simulink model "with_sssc"  (Simulink 7.3)
settings: Solver=FixedStepDiscrete  SolverMode=SingleTasking  StartTime=0.0  StopTime=0.8  FixedStep=Ts  RelTol=1e-3
PreLoadFcn:
  | Ts=1/512/60;
undefined symbols (not defined in the file): DiscIntNeverNeededParam
libraries: powerlib x54, powerlib_extras x38, simulink_extras x2, simulink x1
(part 1 of 7)
Description:
  | Copyright 2008-2009 The MathWorks(TM), Inc.
settings Model: Creator=Giroux/Sybille  LastModifiedBy=Bharath  ExtModeTrigMode=oneshot  ExtModeArmWhenConnect=off  ExtModeAutoUpdateStatusClock=off
settings DataIOCC: InitialState=xInitial_upfc  LimitDataPoints=off  SaveFinalState=on  SaveFormat=Structure  SaveOutput=off  SaveTime=off  SignalLoggingName=sigsOut
settings OptimizationCC: BlockReduction=off  BooleanDataType=off  InitFltsAndDblsToZero=on  EfficientMapNaN2IntZero=off
settings DebuggingCC: SignalResolutionControl=TryResolveAllWithWarning  SolverPrmCheckMsg=none  MultiTaskDSMMsg=warning  MultiTaskCondExecSysMsg=none  StrictBusMsg=None
settings HardwareCC: TargetEndianess=LittleEndian  TargetHWDeviceType=MATLAB Host  ProdEqTarget=off
settings RTWCC: SystemTargetFile=accel.tlc  TemplateMakefile=accel_default_tmf  ProcessScript=accel_make_rtw_hook  IncludeERTFirstTime=on
settings STFCustomTargetCC: SystemTargetFile=accel.tlc

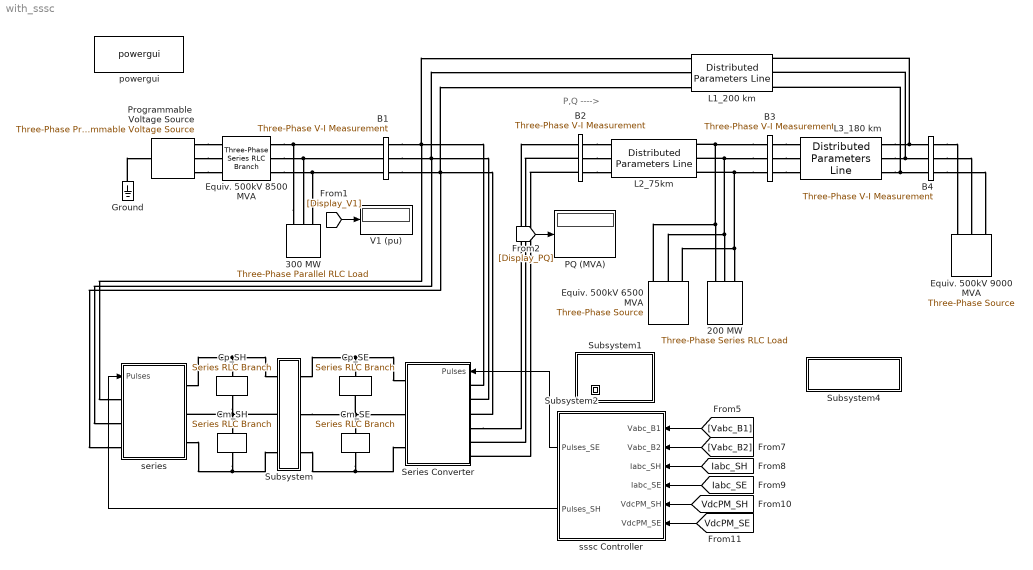
== system with_sssc ==
  note: P,Q
      | ---->
  200 MW : powerlib/Elements/Three-Phase Series RLC Load  DialogController=POWERSYS.PowerSysDialog  PhysicalDomain=powersysdomain  SubClassName=unknown  LeftPortType=p1  RightPortType=p1  LConnTagsString=A|B|C  Configuration=Y (grounded)  NominalVoltage=500e3  NominalFrequency=60  ActivePower=200e6  InductivePower=0  CapacitivePower=0  Measurements=None
  300 MW : powerlib/Elements/Three-Phase Parallel RLC Load  DialogController=POWERSYS.PowerSysDialog  PhysicalDomain=powersysdomain  SubClassName=unknown  LeftPortType=p1  RightPortType=p1  LConnTagsString=A|B|C  Configuration=Y (grounded)  NominalVoltage=500e3  NominalFrequency=60  ActivePower=300e6  InductivePower=0  CapacitivePower=0  Measurements=None
  B1 : powerlib/Measurements/Three-Phase V-I Measurement  DialogController=POWERSYS.PowerSysDialog  SystemSampleTime=-1  VoltageMeasurement=phase-to-ground  SetLabelV=on  LabelV=Vabc_B1  Vpu=on  CurrentMeasurement=yes  SetLabelI=on  LabelI=Iabc_B1  Ipu=on  Pbase=100e6  Vbase=500e3  OutputType=Magnitude  PhasorSimulation=off  PSBequivalent=0
  B2 : powerlib/Measurements/Three-Phase V-I Measurement  DialogController=POWERSYS.PowerSysDialog  SystemSampleTime=-1  VoltageMeasurement=phase-to-ground  SetLabelV=on  LabelV=Vabc_B2  Vpu=on  CurrentMeasurement=yes  SetLabelI=on  LabelI=Iabc_B2  Ipu=on  Pbase=100e6  Vbase=500e3  OutputType=Magnitude  PhasorSimulation=off  PSBequivalent=0
  B3 : powerlib/Measurements/Three-Phase V-I Measurement  DialogController=POWERSYS.PowerSysDialog  SystemSampleTime=-1  VoltageMeasurement=phase-to-ground  SetLabelV=on  LabelV=Vabc_B3  Vpu=on  CurrentMeasurement=yes  SetLabelI=on  LabelI=Iabc_B3  Ipu=on  Pbase=100e6  Vbase=500e3  OutputType=Magnitude  PhasorSimulation=off  PSBequivalent=0
  B4 : powerlib/Measurements/Three-Phase V-I Measurement  DialogController=POWERSYS.PowerSysDialog  SystemSampleTime=-1  VoltageMeasurement=phase-to-ground  SetLabelV=on  LabelV=Vabc_B4  Vpu=on  CurrentMeasurement=no  SetLabelI=on  LabelI=Iabc_B4  Ipu=on  Pbase=100e6  Vbase=500e3  OutputType=Magnitude  PhasorSimulation=off  PSBequivalent=0
  Cm_SE : powerlib/Elements/Series RLC Branch  DialogController=POWERSYS.PowerSysDialog  PhysicalDomain=powersysdomain  SubClassName=unknown  LeftPortType=p1  RightPortType=p1  LConnTagsString=__new0  RConnTagsString=__new0  BranchType=C  Resistance=1.0  Inductance=1.0  SetiL0=off  InitialCurrent=0  Capacitance=2500e-6  Setx0=off  InitialVoltage=0  Measurements=Branch voltage
  Cm_SH : powerlib/Elements/Series RLC Branch  DialogController=POWERSYS.PowerSysDialog  PhysicalDomain=powersysdomain  SubClassName=unknown  LeftPortType=p1  RightPortType=p1  LConnTagsString=__new0  RConnTagsString=__new0  BranchType=C  Resistance=1.0  Inductance=1.0  SetiL0=off  InitialCurrent=0  Capacitance=2500e-6  Setx0=off  InitialVoltage=0  Measurements=Branch voltage
  Cp_SE : powerlib/Elements/Series RLC Branch  DialogController=POWERSYS.PowerSysDialog  PhysicalDomain=powersysdomain  SubClassName=unknown  LeftPortType=p1  RightPortType=p1  LConnTagsString=__new0  RConnTagsString=__new0  BranchType=C  Resistance=1.0  Inductance=1.0  SetiL0=off  InitialCurrent=0  Capacitance=2500e-6  Setx0=off  InitialVoltage=0  Measurements=Branch voltage
  Cp_SH : powerlib/Elements/Series RLC Branch  DialogController=POWERSYS.PowerSysDialog  PhysicalDomain=powersysdomain  SubClassName=unknown  LeftPortType=p1  RightPortType=p1  LConnTagsString=__new0  RConnTagsString=__new0  BranchType=C  Resistance=1.0  Inductance=1.0  SetiL0=off  InitialCurrent=0  Capacitance=2500e-6  Setx0=off  InitialVoltage=0  Measurements=Branch voltage
  Equiv. 500kV 6500 MVA : powerlib/Electrical Sources/Three-Phase Source  DialogController=POWERSYS.PowerSysDialog  SystemSampleTime=-1  Voltage=500e3*1.00  PhaseAngle=9.2-20  Frequency=60  InternalConnection=Yg  SpecifyImpedance=on  Resistance=0.8929  Inductance=16.58e-3  ShortCircuitLevel=6500e6  BaseVoltage=500e3  XRratio=8
  "Equiv. 500kV 8500 MVA " : powerlib/Elements/Three-Phase Series RLC Branch  DialogController=POWERSYS.PowerSysDialog  PhysicalDomain=powersysdomain  SubClassName=unknown  LeftPortType=p1  RightPortType=p1  LConnTagsString=A|B|C  RConnTagsString=A|B|C  BranchType=RL  Resistance=500e3^2/8500e6/10  Inductance=500e3^2/8500e6/(2*pi*60)  Capacitance=1.0  Measurements=None
  Equiv. 500kV 9000 MVA : powerlib/Electrical Sources/Three-Phase Source  DialogController=POWERSYS.PowerSysDialog  SystemSampleTime=-1  Voltage=500e3*0.98  PhaseAngle=9.2-40  Frequency=60  InternalConnection=Yg  SpecifyImpedance=on  Resistance=0.8929  Inductance=16.58e-3  ShortCircuitLevel=9000e6  BaseVoltage=500e3  XRratio=10
  Ground : powerlib/Elements/Ground  DialogController=POWERSYS.PowerSysDialog  PhysicalDomain=powersysdomain  SubClassName=unknown  LeftPortType=p1  RightPortType=p1  LConnTagsString=a
  L1_200 km : powerlib/Elements/Distributed Parameters Line  DialogController=POWERSYS.PowerSysDialog  SystemSampleTime=-1  Phases=3  Frequency=60  Resistance=[0.01273*2 0.3864]  Inductance="[0.9337e-3  4.1264e-3]"  Capacitance=[12.74e-9 7.751e-9]  Length=200  x1=[0 -1.91503257172238e-010 88662.5919859554 -491984.755570925;0.000226216626798297 -1.96856066781718e-010 130246.803325563 -482644.615794399;0.000452433253596594 -2.0077801734948e-010 170884.308682266 -469796.347344288;0.000678649880394891 -2.03240601964242e-010 210279.732135357 -453533.338559508;0.000904866507193188 -2.04225921195624e-010 248146.725904086 -433973.798005056;0.00113108313399149 -2.03726813197136e-010 284210.051682097 -411259.895266619]  x2=[0 -4.21310497148667e-011 -44308.1155382362 -490501.124647627;0.000226216626798297 -3.40783030710814e-011 -2367.02497623426 -492492.598498595;0.000452433253596594 -2.57778564256003e-011 39591.27043571 -490904.363077395;0.000678649880394891 -1.72900420268886e-011 81261.7945424455 -485747.962559677;0.000904866507193188 -8.6765540161297e-012 122341.662870224 -477060.87652341;0.00113108313399149 0 162532.284158993 -464906.247526527]  x3=[0 -1.46364700661107e-012 -25.746556881283 50.0156886130386;0.000226216626798297 -1.43300403371694e-012 -29.9132391703324 47.6408692302741;0.000452433253596594 -1.39194519296574e-012 -33.8624954514681 44.9197695951003;0.000678649880394891 -1.34076892277742e-012 -37.5656203403433 41.8721681684003;0.000904866507193188 -1.27984720065879e-012 -40.9956974720401 38.5202166071091;0.00113108313399149 -1.20962283946473e-012 -44.1277951441326 34.8882787536893]  x4=[0 1.64774342243962e-013 -282.830205301423 -3649.3225183874;0.000226216626798297 4.44601431824641e-014 29.0408455107673 -3660.15087087025;0.000452433253596594 -7.61772168509498e-014 340.700811355867 -3644.37521742502;0.000678649880394891 -1.96260878635252e-013 649.884374799866 -3602.1102242479;0.000904866507193188 -3.1491800753529e-013 954.344218274468 -3533.66309674343;0.00113108313399149 -4.31286137747869e-013 1251.86735882721 -3439.53134658535]  x5=0.00113108313399149  Measurements=None
      settings: AttributesFormatString=\n
  L2_75km : powerlib/Elements/Distributed Parameters Line  DialogController=POWERSYS.PowerSysDialog  SystemSampleTime=-1  Phases=3  Frequency=60  Resistance=[0.01273*2 0.3864]  Inductance="[0.9337e-3  4.1264e-3]"  Capacitance=[12.74e-9 7.751e-9]  Length=75  x1=[0 -3.96693010864502e-010 167104.032532242 -471154.023466305;8.48312350493614e-005 -3.93822769631872e-010 182083.816625282 -465569.925188681;0.000169662470098723 -3.90549776474901e-010 196877.388510213 -459509.701105888;0.000254493705148084 -3.86877378595412e-010 211469.619200078 -452979.548845638;0.000339324940197445 -3.82809331655663e-010 225845.585614131 -445986.146618518;0.000424156175246807 -3.78349795937538e-010 239990.585839268 -438536.646388359]  x2=[0 -6.95097933782165e-012 120539.216595689 -484658.49781756;8.48312350493614e-005 -5.56933300650617e-012 135974.618856574 -480556.412163115;0.000169662470098723 -4.18199106854061e-012 151270.963542253 -475962.874427486;0.000254493705148084 -2.79037232110564e-012 166412.607493587 -470882.582297819;0.000339324940197445 -1.3958999351596e-012 181384.065759707 -465320.731251848;0.000424156175246807 0 196170.027434053 -459283.009244626]  x3=[0 4.40693316305242e-013 -104.937683284578 -46.5969347149227;8.48312350493614e-005 5.09069305089187e-013 -103.394079857967 -49.9285083723259;0.000169662470098723 5.769246824254e-013 -101.744738094624 -53.2090214908851;0.000254493705148084 6.44190054449671e-013 -99.991344731884 -56.4351191783158;0.000339324940197445 7.10796630680306e-013 -98.1356929178462 -59.603502191527;0.000424156175246807 7.76676294368304e-013 -96.1796803775706 -62.7109303106685]  x4=[0 -2.3638910297891e-012 990.165268579737 -3517.07349521636;8.48312350493614e-005 -2.47594506765685e-012 1102.11798749276 -3483.61438329502;0.000169662470098723 -2.58546702328494e-012 1212.94360006623 -3446.59267290369;0.000254493705148084 -2.69234489152335e-012 1322.52876793534 -3406.04622514705;0.000339324940197445 -2.79646937125895e-012 1430.76142130464 -3362.0165057836;0.000424156175246807 -2.89773397719475e-012 1537.53087355877 -3314.54854281976]  x5=0.000424156175246807  Measurements=None
      settings: AttributesFormatString=\n
  L3_180 km : powerlib/Elements/Distributed Parameters Line  DialogController=POWERSYS.PowerSysDialog  SystemSampleTime=-1  Phases=3  Frequency=60  Resistance=[0.01273*2 0.3864]  Inductance="[0.9337e-3  4.1264e-3]"  Capacitance=[12.74e-9 7.751e-9]  Length=180  x1=[0 -1.63454333087056e-011 53455.4761104332 -496554.200785859;0.000203594964118467 -1.31933594894557e-011 91372.9576361359 -490993.426490723;0.000407189928236935 -9.96360043581722e-012 128752.41625445 -482541.581164688;0.000610784892355402 -6.6751736383164e-012 165373.753967862 -471248.431024288;0.000814379856473869 -3.34744203531157e-012 201021.336751836 -457180.472477534;0.00101797482059234 0 235485.264252623 -440420.540579284]  x2=[0 -3.81393443869797e-011 -31539.306669084 -491487.369642364;0.000203594964118467 -3.07845054753967e-011 6239.89303884498 -492458.75575321;0.000407189928236935 -2.32484010169069e-011 43982.3509636315 -490530.442670838;0.000610784892355402 -1.55754051560716e-011 81465.8316926323 -485713.78470223;0.000814379856473869 -7.81069808239367e-012 118469.624724594 -478037.143327535;0.00101797482059234 0 154775.844058816 -467545.720201797]  x3=[0 -5.49396821505064e-013 -34.7229837874336 -492.811835812092;0.000203594964118467 -5.26694805439027e-013 3.16714661805268 -494.023441044943;0.000407189928236935 -5.0089150122538e-013 41.038628208007 -492.326133893369;0.000610784892355402 -4.72138844065877e-013 78.6684658517113 -487.729908453567;0.000814379856473869 -4.40606135563534e-013 115.835087268073 -480.261828253281;0.00101797482059234 -4.06479046839711e-013 152.319647689125 -469.965866896147]  x4=[0 9.1315487305108e-014 -310.779746226165 -3120.093262722;0.000203594964118467 7.3706094431248e-014 -70.6217835689112 -3134.73740246822;0.000407189928236935 5.56627048011912e-014 169.952014783101 -3130.92355885908;0.000610784892355402 3.72915616317389e-014 409.52510045736 -3108.674188596;0.000814379856473869 1.87008380204443e-014 646.686817484955 -3068.12030058126;0.00101797482059234 1.26217744835362e-029 880.040708535207 -3009.50068451039]  x5=0.00101797482059234  Measurements=None
      settings: AttributesFormatString=\n
  PQ (MVA) : Display
      settings: Format=bank  SampleTime=Ts*100
  Programmable  Voltage Source : powerlib/Electrical Sources/Three-Phase Programmable Voltage Source  DialogController=POWERSYS.PowerSysDialog  SystemSampleTime=-1  PositiveSequence="[500e3*1.0491 9.2  60]"  VariationEntity=None  VariationType=Modulation  VariationStep=-0.3  VariationRate=0.5  VariationMagnitude=0.4  VariationFrequency=2  VariationTiming=[0.1 1.2]  VariationPhaseA=off  Amplitudes="[1  0.8  1.2  1.0 ]"  TimeValues=[0 0.1 0.25 0.4]  HarmonicGeneration=off  HarmonicA=[3 0.2 -25 0]  HarmonicB="[2 0.15  35 2]"  Timing="[0.1  0.6]"
  Series Converter : Subsystem
  Subsystem : Subsystem
      mask Display: disp('Sw')
  Subsystem1 : Subsystem  mask(UPFC GUI){OpMode=SSSC (Voltage Injection), Par_VarControl=[0.3  0.5  +0.8  -0.8 ], Par_Vref=[ 1  1.005  0.3 *100], Par_SSSC=[ 0.0  0.08  0.3  ], Par_UPFC_Pref=[  +8.7  +10   0.25  ], Par_UPFC_Qref=[  -0.6  +0.7  0.5  ]}
      mask prompts: OpMode "Operation Mode:"; Par_VarControl "STATCOM (Qref): [T1 T2 Q1 Q2]"; Par_Vref "STATCOM Vref (pu): [ Initial   Final  StepTime ]"; Par_SSSC "SSSC Votage Injection (pu): [ Initial  Final  StepTime ]"; Par_UPFC_Pref "UPFC Pref (pu): [ Initial  Final  StepTime ]"; Par_UPFC_Qref "UPFC Qref (pu): [ Initial  Final  StepTime ]"
      mask StyleString: popup(STATCOM (Var Control)|STATCOM (Voltage Control)|SSSC (Voltage Injection)|STATCOM  (Voltage Control) + SSSC (Voltage Injection)|UPFC  (Power Flow Control)),edit,edit,edit,edit,edit
      mask Display: disp('SSSC\nGUI')
  Subsystem2 : Subsystem  mask(UPFC GUI){OpMode=SSSC (Voltage Injection), Par_VarControl=[0.05 0.15 -0.5 0.5]*100, Par_Vref=[ 1  1.005  0.1*100 ], Par_SSSC=[ 0.0  0.08 0.1*100 ], Par_UPFC_Pref=[  8.7  10  0.1*100 ], Par_UPFC_Qref=[  -0.6  +0.5  0.1*100 ]}
      mask prompts: OpMode "Operation Mode:"; Par_VarControl "STATCOM (Qref): [T1 T2 Q1 Q2]"; Par_Vref "STATCOM Vref (pu): [ Initial   Final  StepTime ]"; Par_SSSC "SSSC Votage Injection (pu): [ Initial  Final  StepTime ]"; Par_UPFC_Pref "UPFC Pref (pu): [ Initial  Final  StepTime ]"; Par_UPFC_Qref "UPFC Qref (pu): [ Initial  Final  StepTime ]"
      settings: OpenFcn=openfig('power_upfc_gto48p_PQregion.fig');
      mask StyleString: popup(STATCOM (Var Control)|STATCOM (Voltage Control)|SSSC (Voltage Injection)|STATCOM  (Voltage Control) + SSSC (Voltage Injection)|UPFC  (Power Flow Control)),edit,edit,edit,edit,edit
      mask Display: disp('Show UPFC\nControllable Region')
  Subsystem4 : Subsystem
      mask Display: disp('Show Scopes')
  V1 (pu) : Display
      settings: Format=bank  SampleTime=Ts*100
  powergui : powerlib/powergui  Priority=2  SystemSampleTime=-1  SimulationMode=Discrete  SampleTime=Ts  frequency=60  SPID=off  DisableSnubberDevices=off  DisableRonSwitches=off  DisableVfSwitches=off  SwTol=0  Interpol=off  frequencyindice=60  echomessages=off  HookPort=off  DisplayEquations=off  FunctionMessages=off  EnableUseOfTLC=off  x0status=blocks  RestoreLinks=yes  Frange=[0:2:500]  Ylog=off  Xlog=on  ShowGrid=off  save=off  variable=ZData  ZoomFFT=on  StartTime=0.0  cycles=1  DisplayStyle=1  fundamental=60  FreqAxis=off  MaxFrequency=1000  frequencyindicesteady=1  RmsSteady=1  display=off  Ts=0  methode=off
  series : Subsystem
  sssc Controller : Subsystem
  wires:
  [Vabc_B1] -> sssc Controller/1(Vabc_B1)
  [Vabc_B2] -> sssc Controller/2(Vabc_B2)
  [Iabc_SH] -> sssc Controller/3("Iabc_SH ")
  [Iabc_SE] -> sssc Controller/4(Iabc_SE)
  [VdcPM_SH] -> sssc Controller/5("VdcPM_SH ")
  [VdcPM_SE] -> sssc Controller/6(VdcPM_SE)
  sssc Controller/2(Pulses_SH) -> series/1(Pulses)
  sssc Controller/1(Pulses_SE) -> Series Converter/1(Pulses)
  [Display_V1] -> V1 (pu)/1
  [Display_PQ] -> PQ (MVA)/1
  connections:
  Ground/LConn1 -- Programmable  Voltage Source/LConn1
  Programmable  Voltage Source/RConn1 -- "Equiv. 500kV 8500 MVA "/LConn1
  Programmable  Voltage Source/RConn2 -- "Equiv. 500kV 8500 MVA "/LConn2
  Programmable  Voltage Source/RConn3 -- "Equiv. 500kV 8500 MVA "/LConn3
  Subsystem/LConn2 -- series/RConn2 -- Cp_SH/RConn1 -- Cm_SH/LConn1
  Subsystem/RConn3 -- Series Converter/RConn3 -- Cm_SE/RConn1
  Subsystem/RConn1 -- Series Converter/RConn1 -- Cp_SE/LConn1
  B3/LConn1 -- 200 MW/LConn1 -- Equiv. 500kV 6500 MVA/RConn1 -- L2_75km/RConn1
  B3/LConn2 -- 200 MW/LConn2 -- Equiv. 500kV 6500 MVA/RConn2 -- L2_75km/RConn2
  B3/LConn3 -- 200 MW/LConn3 -- Equiv. 500kV 6500 MVA/RConn3 -- L2_75km/RConn3
  "Equiv. 500kV 8500 MVA "/RConn2 -- 300 MW/LConn2 -- B1/LConn2
  "Equiv. 500kV 8500 MVA "/RConn3 -- 300 MW/LConn3 -- B1/LConn3
  B2/RConn1 -- L2_75km/LConn1
  B2/RConn2 -- L2_75km/LConn2
  B2/RConn3 -- L2_75km/LConn3
  B3/RConn1 -- L3_180 km/LConn1
  B3/RConn2 -- L3_180 km/LConn2
  B3/RConn3 -- L3_180 km/LConn3
  300 MW/LConn1 -- "Equiv. 500kV 8500 MVA "/RConn1 -- B1/LConn1
  L3_180 km/RConn1 -- B4/LConn1 -- L1_200 km/RConn1
  L3_180 km/RConn2 -- B4/LConn2 -- L1_200 km/RConn2
  L3_180 km/RConn3 -- B4/LConn3 -- L1_200 km/RConn3
  B4/RConn1 -- Equiv. 500kV 9000 MVA/RConn1
  B4/RConn2 -- Equiv. 500kV 9000 MVA/RConn2
  B4/RConn3 -- Equiv. 500kV 9000 MVA/RConn3
  series/LConn1 -- B1/RConn1 -- L1_200 km/LConn1 -- Series Converter/LConn1
  Series Converter/LConn2 -- B1/RConn2 -- L1_200 km/LConn2 -- series/LConn2
  series/LConn3 -- B1/RConn3 -- L1_200 km/LConn3 -- Series Converter/LConn3
  Series Converter/LConn4 -- B2/LConn1
  B2/LConn2 -- Series Converter/LConn5
  B2/LConn3 -- Series Converter/LConn6
  Subsystem/RConn2 -- Series Converter/RConn2 -- Cm_SE/LConn1 -- Cp_SE/RConn1
  series/RConn1 -- Subsystem/LConn1 -- Cp_SH/LConn1
  series/RConn3 -- Subsystem/LConn3 -- Cm_SH/RConn1

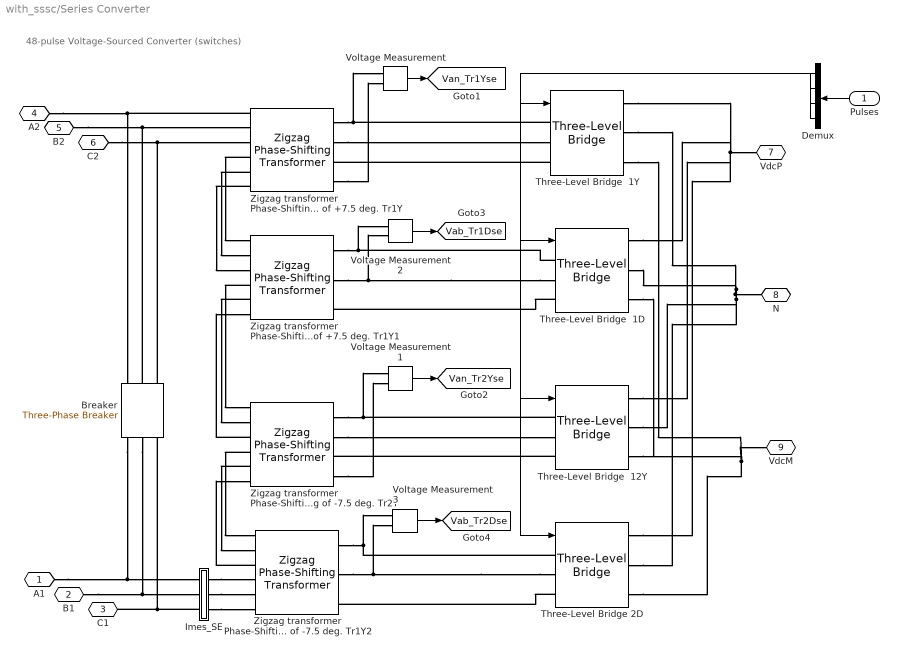
== system with_sssc/Series Converter ==
  note: 48-pulse Voltage-Sourced Converter
      | (switches)
  Pulses : Inport  PortDimensions=48  OutDataType=sfix(16)  OutScaling=2^0
  Breaker : powerlib/Elements/Three-Phase Breaker  DialogController=POWERSYS.PowerSysDialog  SystemSampleTime=-1  InitialState=closed  SwitchA=on  SwitchB=on  SwitchC=on  SwitchTimes=[ 0]  External=off  BreakerResistance=0.0001  SnubberResistance=1e6  SnubberCapacitance=inf  Measurements=None
      settings: AttributesFormatString=\n
  Demux : Demux  Outputs=[12 12 12 12]
  Imes_SE : Subsystem
  Three-Level Bridge  12Y : powerlib/Power Electronics/Three-Level Bridge  DialogController=POWERSYS.PowerSysDialog  SystemSampleTime=-1  Arms=3  SnubberResistance=1e5  SbubberCapacitance=inf  Device=GTO / Diodes  Ron=1e-4  ForwardVoltages="[  0  0  ]"  Measurements=None
  Three-Level Bridge  1D : powerlib/Power Electronics/Three-Level Bridge  DialogController=POWERSYS.PowerSysDialog  SystemSampleTime=-1  Arms=3  SnubberResistance=1e5  SbubberCapacitance=inf  Device=GTO / Diodes  Ron=1e-4  ForwardVoltages="[  0  0  ]"  Measurements=None
  Three-Level Bridge  1Y : powerlib/Power Electronics/Three-Level Bridge  DialogController=POWERSYS.PowerSysDialog  SystemSampleTime=-1  Arms=3  SnubberResistance=1e5  SbubberCapacitance=inf  Device=GTO / Diodes  Ron=1e-4  ForwardVoltages="[  0  0  ]"  Measurements=None
  Three-Level Bridge 2D : powerlib/Power Electronics/Three-Level Bridge  DialogController=POWERSYS.PowerSysDialog  SystemSampleTime=-1  Arms=3  SnubberResistance=1e5  SbubberCapacitance=inf  Device=GTO / Diodes  Ron=1e-4  ForwardVoltages="[  0  0  ]"  Measurements=None
  Voltage Measurement{,1..3} (4 alike) : powerlib/Measurements/Voltage Measurement  Tag=PoWeRsYsTeMmEaSuReMeNt  DialogController=POWERSYS.PowerSysDialog  SystemSampleTime=-1  PhasorSimulation=off  OutputType=Magnitude  PSBequivalent=0
  Zigzag transformer Phase-Shifting of +7.5 deg. Tr1Y : powerlib/Elements/Zigzag Phase-Shifting Transformer  DialogController=POWERSYS.PowerSysDialog  SystemSampleTime=-1  SecondaryConnection=Yn  UNITS=pu  NominalPower=[ 100e6/4 60]  PrimaryVoltage=12.5e3  SecondaryVoltage="[ 12.5e3  +7.5]"  Winding1=[ 0.05/30 0.05 ]  Winding2=[ 0.05/30 0.05 ]  Winding3=[ 0.05/30 0.05 ]  SetSaturation=off  RmLm=[ 500 500 ]  Rm=500  Saturation=[ 0,0 ; 0.0024,1.2 ; 1.0,1.52 ]  SetInitialFlux=off  Measurements=None  InitialFluxes=[0,0,0]  MoreParameters=off  BreakLoop=off  DataType=off
      settings: AttributesFormatString=\n
  Zigzag transformer Phase-Shifting of +7.5 deg. Tr1Y1 : powerlib/Elements/Zigzag Phase-Shifting Transformer  DialogController=POWERSYS.PowerSysDialog  SystemSampleTime=-1  SecondaryConnection=Delta D1(-30 deg.)  UNITS=pu  NominalPower=[ 100e6/4 60]  PrimaryVoltage=12.5e3  SecondaryVoltage="[ 12.5e3  +7.5]"  Winding1=[ 0.05/30 0.05 ]  Winding2=[ 0.05/30 0.05 ]  Winding3=[ 0.05/30 0.05 ]  SetSaturation=off  RmLm=[ 500 500 ]  Rm=500  Saturation=[ 0,0 ; 0.0024,1.2 ; 1.0,1.52 ]  SetInitialFlux=off  Measurements=None  InitialFluxes=[0,0,0]  MoreParameters=off  BreakLoop=off  DataType=off
      settings: AttributesFormatString=\n
  Zigzag transformer Phase-Shifting of -7.5 deg. Tr1Y2 : powerlib/Elements/Zigzag Phase-Shifting Transformer  DialogController=POWERSYS.PowerSysDialog  SystemSampleTime=-1  SecondaryConnection=Delta D1(-30 deg.)  UNITS=pu  NominalPower=[ 100e6/4 60]  PrimaryVoltage=12.5e3  SecondaryVoltage="[ 12.5e3  -7.5]"  Winding1=[ 0.05/30 0.05 ]  Winding2=[ 0.05/30 0.05 ]  Winding3=[ 0.05/30 0.05 ]  SetSaturation=off  RmLm=[ 500 500 ]  Rm=500  Saturation=[ 0,0 ; 0.0024,1.2 ; 1.0,1.52 ]  SetInitialFlux=off  Measurements=None  InitialFluxes=[0,0,0]  MoreParameters=off  BreakLoop=off  DataType=off
      settings: AttributesFormatString=\n
  Zigzag transformer Phase-Shifting of -7.5 deg. Tr2Y : powerlib/Elements/Zigzag Phase-Shifting Transformer  DialogController=POWERSYS.PowerSysDialog  SystemSampleTime=-1  SecondaryConnection=Yn  UNITS=pu  NominalPower=[ 100e6/4 60]  PrimaryVoltage=12.5e3  SecondaryVoltage="[ 12.5e3  -7.5]"  Winding1=[ 0.05/30 0.05 ]  Winding2=[ 0.05/30 0.05 ]  Winding3=[ 0.05/30 0.05 ]  SetSaturation=off  RmLm=[ 500 500 ]  Rm=500  Saturation=[ 0,0 ; 0.0024,1.2 ; 1.0,1.52 ]  SetInitialFlux=off  Measurements=None  InitialFluxes=[0,0,0]  MoreParameters=off  BreakLoop=off  DataType=off
      settings: AttributesFormatString=\n
  "A1 " : PMIOPort  Port=1  Side=Left
  "B1 " : PMIOPort  Port=2  Side=Left
  C1 : PMIOPort  Port=3  Side=Left
  "A2 " : PMIOPort  Port=4  Side=Left
  "B2 " : PMIOPort  Port=5  Side=Left
  "C2 " : PMIOPort  Port=6  Side=Left
  VdcP : PMIOPort  Port=7  Side=Right
  N : PMIOPort  Port=8  Side=Right
  VdcM : PMIOPort  Port=9  Side=Right
  tag scope: Vab_Tr1Dse=global, Vab_Tr2Dse=global, Van_Tr1Yse=global, Van_Tr2Yse=global
  wires:
  Pulses/1 -> Demux/1
  Demux/4 -> Three-Level Bridge 2D/1
  Demux/3 -> Three-Level Bridge  12Y/1
  Demux/2 -> Three-Level Bridge  1D/1
  Demux/1 -> Three-Level Bridge  1Y/1
  Voltage Measurement3/1 -> [Vab_Tr2Dse]
  Voltage Measurement2/1 -> [Vab_Tr1Dse]
  Voltage Measurement1/1 -> [Van_Tr2Yse]
  Voltage Measurement/1 -> [Van_Tr1Yse]
  connections:
  Zigzag transformer Phase-Shifting of -7.5 deg. Tr2Y/RConn4 -- Voltage Measurement1/LConn2
  Zigzag transformer Phase-Shifting of +7.5 deg. Tr1Y/RConn4 -- Voltage Measurement/LConn2
  Three-Level Bridge  1Y/RConn3 -- VdcM/RConn1 -- Three-Level Bridge  1D/RConn3 -- Three-Level Bridge 2D/RConn3 -- Three-Level Bridge  12Y/RConn3
  Three-Level Bridge  12Y/RConn2 -- Three-Level Bridge  1D/RConn2 -- Three-Level Bridge  1Y/RConn2 -- N/RConn1 -- Three-Level Bridge 2D/RConn2
  Three-Level Bridge  1Y/RConn1 -- VdcP/RConn1 -- Three-Level Bridge  1D/RConn1 -- Three-Level Bridge  12Y/RConn1 -- Three-Level Bridge 2D/RConn1
  Three-Level Bridge  1D/LConn1 -- Zigzag transformer Phase-Shifting of +7.5 deg. Tr1Y1/RConn1 -- Voltage Measurement2/LConn1
  Imes_SE/RConn1 -- Zigzag transformer Phase-Shifting of -7.5 deg. Tr1Y2/LConn4
  Imes_SE/RConn2 -- Zigzag transformer Phase-Shifting of -7.5 deg. Tr1Y2/LConn5
  Imes_SE/RConn3 -- Zigzag transformer Phase-Shifting of -7.5 deg. Tr1Y2/LConn6
  "A1 "/RConn1 -- Imes_SE/LConn1 -- Breaker/RConn1
  Zigzag transformer Phase-Shifting of +7.5 deg. Tr1Y/LConn4 -- Zigzag transformer Phase-Shifting of +7.5 deg. Tr1Y1/LConn1
  Zigzag transformer Phase-Shifting of +7.5 deg. Tr1Y/LConn5 -- Zigzag transformer Phase-Shifting of +7.5 deg. Tr1Y1/LConn2
  Zigzag transformer Phase-Shifting of +7.5 deg. Tr1Y/LConn6 -- Zigzag transformer Phase-Shifting of +7.5 deg. Tr1Y1/LConn3
  Zigzag transformer Phase-Shifting of +7.5 deg. Tr1Y1/LConn4 -- Zigzag transformer Phase-Shifting of -7.5 deg. Tr2Y/LConn1
  Zigzag transformer Phase-Shifting of +7.5 deg. Tr1Y1/LConn5 -- Zigzag transformer Phase-Shifting of -7.5 deg. Tr2Y/LConn2
  Zigzag transformer Phase-Shifting of -7.5 deg. Tr2Y/LConn3 -- Zigzag transformer Phase-Shifting of +7.5 deg. Tr1Y1/LConn6
  Zigzag transformer Phase-Shifting of -7.5 deg. Tr2Y/LConn4 -- Zigzag transformer Phase-Shifting of -7.5 deg. Tr1Y2/LConn1
  Zigzag transformer Phase-Shifting of -7.5 deg. Tr2Y/LConn5 -- Zigzag transformer Phase-Shifting of -7.5 deg. Tr1Y2/LConn2
  Zigzag transformer Phase-Shifting of -7.5 deg. Tr1Y2/LConn3 -- Zigzag transformer Phase-Shifting of -7.5 deg. Tr2Y/LConn6
  Three-Level Bridge  1Y/LConn1 -- Zigzag transformer Phase-Shifting of +7.5 deg. Tr1Y/RConn1 -- Voltage Measurement/LConn1
  Three-Level Bridge  12Y/LConn1 -- Zigzag transformer Phase-Shifting of -7.5 deg. Tr2Y/RConn1 -- Voltage Measurement1/LConn1
  Three-Level Bridge 2D/LConn1 -- Zigzag transformer Phase-Shifting of -7.5 deg. Tr1Y2/RConn1 -- Voltage Measurement3/LConn1
  Imes_SE/LConn3 -- Breaker/RConn3 -- C1/RConn1
  "B1 "/RConn1 -- Imes_SE/LConn2 -- Breaker/RConn2
  Breaker/LConn3 -- Zigzag transformer Phase-Shifting of +7.5 deg. Tr1Y/LConn3 -- "C2 "/RConn1
  Breaker/LConn2 -- Zigzag transformer Phase-Shifting of +7.5 deg. Tr1Y/LConn2 -- "B2 "/RConn1
  Zigzag transformer Phase-Shifting of +7.5 deg. Tr1Y/LConn1 -- Breaker/LConn1 -- "A2 "/RConn1
  Three-Level Bridge  1Y/LConn3 -- Zigzag transformer Phase-Shifting of +7.5 deg. Tr1Y/RConn3
  Zigzag transformer Phase-Shifting of +7.5 deg. Tr1Y/RConn2 -- Three-Level Bridge  1Y/LConn2
  Three-Level Bridge  1D/LConn2 -- Zigzag transformer Phase-Shifting of +7.5 deg. Tr1Y1/RConn2 -- Voltage Measurement2/LConn2
  Three-Level Bridge  1D/LConn3 -- Zigzag transformer Phase-Shifting of +7.5 deg. Tr1Y1/RConn3
  Zigzag transformer Phase-Shifting of -7.5 deg. Tr2Y/RConn2 -- Three-Level Bridge  12Y/LConn2
  Three-Level Bridge  12Y/LConn3 -- Zigzag transformer Phase-Shifting of -7.5 deg. Tr2Y/RConn3
  Three-Level Bridge 2D/LConn2 -- Zigzag transformer Phase-Shifting of -7.5 deg. Tr1Y2/RConn2 -- Voltage Measurement3/LConn2
  Three-Level Bridge 2D/LConn3 -- Zigzag transformer Phase-Shifting of -7.5 deg. Tr1Y2/RConn3

== system with_sssc/Subsystem ==
  Sw1 : powerlib/Power Electronics/Ideal Switch  DialogController=POWERSYS.PowerSysDialog  SystemSampleTime=-1  Ron=0.0001  Lon=0  IC=0  Rs=inf  Cs=0  Measurements=off
      settings: AttributesFormatString=\n
  Sw2 : powerlib/Power Electronics/Ideal Switch  DialogController=POWERSYS.PowerSysDialog  SystemSampleTime=-1  Ron=0.0001  Lon=0  IC=0  Rs=inf  Cs=0  Measurements=off
      settings: AttributesFormatString=\n
  "VdcP " : PMIOPort  Port=1  Side=Left
  "N " : PMIOPort  Port=2  Side=Left
  "VdcM " : PMIOPort  Port=3  Side=Left
  " VdcP" : PMIOPort  Port=4  Side=Right
  " N" : PMIOPort  Port=5  Side=Right
  " VdcM" : PMIOPort  Port=6  Side=Right
  wires:
  [Sw_On] -> Sw1/1, Sw2/1
  connections:
  " VdcP"/RConn1 -- Sw1/RConn1
  "VdcP "/RConn1 -- Sw1/LConn1
  " VdcM"/RConn1 -- Sw2/RConn1
  "VdcM "/RConn1 -- Sw2/LConn1
  "N "/RConn1 -- " N"/RConn1

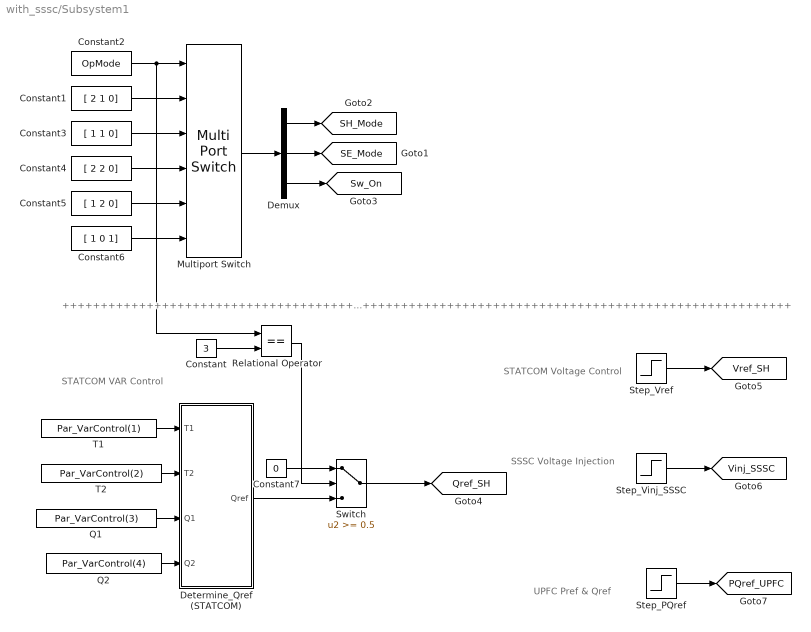
== system with_sssc/Subsystem1 ==
  note: +++++++++++++++++++++++++++++++++++++++++++++++++++++++++++++++++++++++++++++++++++++++++++++++++++++++++++++++++++
  note: STATCOM
      | VAR Control
  note: STATCOM
      | Voltage Control
  note: SSSC
      | Voltage Injection
  note: UPFC
      | Pref & Qref
  Constant : Constant  Value=3  OutDataType=sfix(16)  OutScaling=2^0
  Constant1 : Constant  Value=[ 2 1 0]  OutDataType=sfix(16)  OutScaling=2^0
  Constant2 : Constant  Value=OpMode  OutDataType=sfix(16)  OutScaling=2^0
  Constant3 : Constant  Value=[ 1 1 0]  OutDataType=sfix(16)  OutScaling=2^0
  Constant4 : Constant  Value=[ 2 2 0]  OutDataType=sfix(16)  OutScaling=2^0
  Constant5 : Constant  Value=[ 1 2 0]  OutDataType=sfix(16)  OutScaling=2^0
  Constant6 : Constant  Value=[ 1 0 1]  OutDataType=sfix(16)  OutScaling=2^0
  Constant7 : Constant  Value=0  OutDataType=sfix(16)  OutScaling=2^0
  Demux : Demux  Outputs=3
  Determine_Qref (STATCOM) : Subsystem
  Multiport Switch : MultiPortSwitch  Inputs=5  OutDataType=sfix(16)  OutScaling=2^0  SaturateOnIntegerOverflow=on
  Q1 : Constant  Value=Par_VarControl(3)  OutDataType=sfix(16)  OutScaling=2^0
  Q2 : Constant  Value=Par_VarControl(4)  OutDataType=sfix(16)  OutScaling=2^0
  Relational Operator : RelationalOperator  Operator===
  Step_PQref : Step  Time=[Par_UPFC_Pref(3) Par_UPFC_Qref(3) ]  Before=[Par_UPFC_Pref(1) Par_UPFC_Qref(1) ]  After=[Par_UPFC_Pref(2) Par_UPFC_Qref(2) ]  SampleTime=0
  Step_Vinj_SSSC : Step  Time=Par_SSSC(3)  Before=Par_SSSC(1)  After=Par_SSSC(2)  SampleTime=0
  Step_Vref : Step  Time=Par_Vref(3)  Before=Par_Vref(1)  After=Par_Vref(2)  SampleTime=0
  Switch : Switch  Threshold=0.5  OutDataType=sfix(16)  OutScaling=2^0  SaturateOnIntegerOverflow=on
  T1 : Constant  Value=Par_VarControl(1)  OutDataType=sfix(16)  OutScaling=2^0
  T2 : Constant  Value=Par_VarControl(2)  OutDataType=sfix(16)  OutScaling=2^0
  tag scope: PQref_UPFC=global, Qref_SH=global, SE_Mode=global, SH_Mode=global, Sw_On=global, Vinj_SSSC=global, Vref_SH=global
  wires:
  Constant2/1 -> Multiport Switch/1, Relational Operator/1
  Multiport Switch/1 -> Demux/1
  Demux/1 -> [SH_Mode]
  Demux/2 -> [SE_Mode]
  Demux/3 -> [Sw_On]
  Constant1/1 -> Multiport Switch/2
  Constant6/1 -> Multiport Switch/6
  Constant5/1 -> Multiport Switch/5
  Constant3/1 -> Multiport Switch/3
  Constant4/1 -> Multiport Switch/4
  T1/1 -> Determine_Qref (STATCOM)/1(T1)
  T2/1 -> Determine_Qref (STATCOM)/2(T2)
  Q1/1 -> Determine_Qref (STATCOM)/3(Q1)
  Q2/1 -> Determine_Qref (STATCOM)/4(Q2)
  Determine_Qref (STATCOM)/1(Qref) -> Switch/3
  Switch/1 -> [Qref_SH]
  Constant/1 -> Relational Operator/2
  Relational Operator/1 -> Switch/2
  Constant7/1 -> Switch/1
  Step_Vref/1 -> [Vref_SH]
  Step_PQref/1 -> [PQref_UPFC]
  Step_Vinj_SSSC/1 -> [Vinj_SSSC]

== system with_sssc/Subsystem2 ==

== system with_sssc/Subsystem4 ==
  Data Acquisition : Subsystem
  SSSC : Scope  NumInputPorts=6
      settings: TimeRange=0.8  YMin=-0.03~-10~0~19300~650~-70  YMax=0.03~10~0.015~19345~1000~0  SaveName=SSSC1  SampleInput=on  SampleTime=Ts*2
  SSSC1 : Scope
      settings: TimeRange=0.8  YMin=-12  YMax=12  SaveName=SSSC  SampleInput=on  SampleTime=Ts*2
  SSSC2 : Scope
      settings: TimeRange=0.8  YMin=-0.09  YMax=0.09  SaveName=SSSC2  SampleInput=on  SampleTime=Ts*2
  SSSC3 : Scope
      settings: TimeRange=0.8  YMin=14902.5  YMax=14950  SaveName=SSSC3  SampleInput=on  SampleTime=Ts*2
  SSSC4 : Scope  NumInputPorts=4
      settings: TimeRange=0.8  YMin=-0.03~-10~0~19300  YMax=0.03~10~0.015~19345  SaveName=SSSC4  SampleInput=on  SampleTime=Ts*2
  wires:
  Data Acquisition/6(Iabc_SE) -> SSSC/2, SSSC1/1  "Iabc (pu)"
  Data Acquisition/5(Vinj_SE) -> SSSC/1, SSSC2/1  "Vinj (pu)"
  Data Acquisition/7(Vmeas_Vref_SSSC) -> SSSC/3  "Mag_Vinj  / Vref (pu)"
  Data Acquisition/8(Vdc_SE) -> SSSC/4, SSSC3/1  "Vdc"
  Data Acquisition/9(P_L123) -> SSSC/5  "P L1 L2 L3 (MW)"
  Data Acquisition/10(Q_L123) -> SSSC/6  "Q L1 L2 L3 (Mvar)"
  Data Acquisition/1(VsVpI_SH) -> SSSC4/1  "Vs Vp Ip (pu)"
  Data Acquisition/2(Vdc_SH) -> SSSC4/2  "Vdc (V)"
  Data Acquisition/3(Q_Qref_SH) -> SSSC4/3  "Q Qref (pu)"
  Data Acquisition/4(VmeasVref_SH) -> SSSC4/4  "Vmeas Vref (pu)"

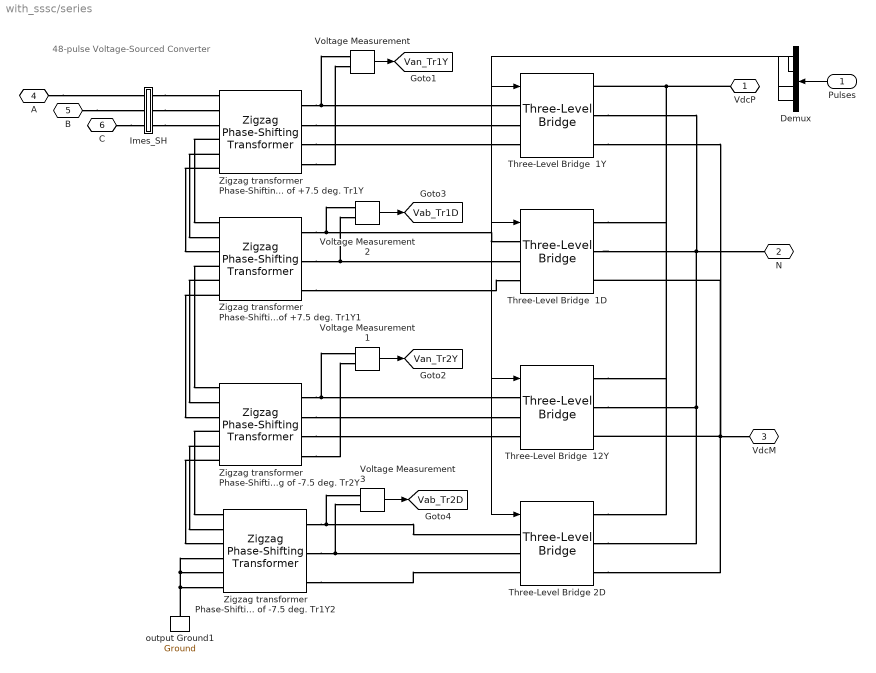
== system with_sssc/series ==
  note: 48-pulse Voltage-Sourced Converter
  Pulses : Inport  PortDimensions=48  OutDataType=sfix(16)  OutScaling=2^0
  Demux : Demux  Outputs=[12 12 12 12]
  Imes_SH : Subsystem
  Three-Level Bridge  12Y : powerlib/Power Electronics/Three-Level Bridge  DialogController=POWERSYS.PowerSysDialog  SystemSampleTime=-1  Arms=3  SnubberResistance=1e5  SbubberCapacitance=inf  Device=GTO / Diodes  Ron=1e-4  ForwardVoltages="[  0  0  ]"  Measurements=None
  Three-Level Bridge  1D : powerlib/Power Electronics/Three-Level Bridge  DialogController=POWERSYS.PowerSysDialog  SystemSampleTime=-1  Arms=3  SnubberResistance=1e5  SbubberCapacitance=inf  Device=GTO / Diodes  Ron=1e-4  ForwardVoltages="[  0  0  ]"  Measurements=None
  Three-Level Bridge  1Y : powerlib/Power Electronics/Three-Level Bridge  DialogController=POWERSYS.PowerSysDialog  SystemSampleTime=-1  Arms=3  SnubberResistance=1e5  SbubberCapacitance=inf  Device=GTO / Diodes  Ron=1e-4  ForwardVoltages="[  0  0  ]"  Measurements=None
  Three-Level Bridge 2D : powerlib/Power Electronics/Three-Level Bridge  DialogController=POWERSYS.PowerSysDialog  SystemSampleTime=-1  Arms=3  SnubberResistance=1e5  SbubberCapacitance=inf  Device=GTO / Diodes  Ron=1e-4  ForwardVoltages="[  0  0  ]"  Measurements=None
  Voltage Measurement{,1..3} (4 alike) : powerlib/Measurements/Voltage Measurement  Tag=PoWeRsYsTeMmEaSuReMeNt  DialogController=POWERSYS.PowerSysDialog  SystemSampleTime=-1  PhasorSimulation=off  OutputType=Magnitude  PSBequivalent=0
  Zigzag transformer Phase-Shifting of +7.5 deg. Tr1Y : powerlib/Elements/Zigzag Phase-Shifting Transformer  DialogController=POWERSYS.PowerSysDialog  SystemSampleTime=-1  SecondaryConnection=Yn  UNITS=pu  NominalPower=[ 100e6/4 60]  PrimaryVoltage=500e3/4  SecondaryVoltage="[ 15e3  +7.5]"  Winding1=[ 0.05/30 0.05 ]  Winding2=[ 0.05/30 0.05 ]  Winding3=[ 0.05/30 0.05 ]  SetSaturation=off  RmLm=[ 500 500 ]  Rm=500  Saturation=[ 0,0 ; 0.0024,1.2 ; 1.0,1.52 ]  SetInitialFlux=off  Measurements=None  InitialFluxes=[0,0,0]  MoreParameters=off  BreakLoop=off  DataType=off
      settings: AttributesFormatString=\n
  Zigzag transformer Phase-Shifting of +7.5 deg. Tr1Y1 : powerlib/Elements/Zigzag Phase-Shifting Transformer  DialogController=POWERSYS.PowerSysDialog  SystemSampleTime=-1  SecondaryConnection=Delta D1(-30 deg.)  UNITS=pu  NominalPower=[ 100e6/4 60]  PrimaryVoltage=500e3/4  SecondaryVoltage="[ 15e3  +7.5]"  Winding1=[ 0.05/30 0.05 ]  Winding2=[ 0.05/30 0.05 ]  Winding3=[ 0.05/30 0.05 ]  SetSaturation=off  RmLm=[ 500 500 ]  Rm=500  Saturation=[ 0,0 ; 0.0024,1.2 ; 1.0,1.52 ]  SetInitialFlux=off  Measurements=None  InitialFluxes=[0,0,0]  MoreParameters=off  BreakLoop=off  DataType=off
      settings: AttributesFormatString=\n
  Zigzag transformer Phase-Shifting of -7.5 deg. Tr1Y2 : powerlib/Elements/Zigzag Phase-Shifting Transformer  DialogController=POWERSYS.PowerSysDialog  SystemSampleTime=-1  SecondaryConnection=Delta D1(-30 deg.)  UNITS=pu  NominalPower=[ 100e6/4 60]  PrimaryVoltage=500e3/4  SecondaryVoltage="[ 15e3  -7.5]"  Winding1=[ 0.05/30 0.05 ]  Winding2=[ 0.05/30 0.05 ]  Winding3=[ 0.05/30 0.05 ]  SetSaturation=off  RmLm=[ 500 500 ]  Rm=500  Saturation=[ 0,0 ; 0.0024,1.2 ; 1.0,1.52 ]  SetInitialFlux=off  Measurements=None  InitialFluxes=[0,0,0]  MoreParameters=off  BreakLoop=off  DataType=off
      settings: AttributesFormatString=\n
  Zigzag transformer Phase-Shifting of -7.5 deg. Tr2Y : powerlib/Elements/Zigzag Phase-Shifting Transformer  DialogController=POWERSYS.PowerSysDialog  SystemSampleTime=-1  SecondaryConnection=Yn  UNITS=pu  NominalPower=[ 100e6/4 60]  PrimaryVoltage=500e3/4  SecondaryVoltage="[ 15e3  -7.5]"  Winding1=[ 0.05/30 0.05 ]  Winding2=[ 0.05/30 0.05 ]  Winding3=[ 0.05/30 0.05 ]  SetSaturation=off  RmLm=[ 500 500 ]  Rm=500  Saturation=[ 0,0 ; 0.0024,1.2 ; 1.0,1.52 ]  SetInitialFlux=off  Measurements=None  InitialFluxes=[0,0,0]  MoreParameters=off  BreakLoop=off  DataType=off
      settings: AttributesFormatString=\n
  output Ground1 : powerlib/Elements/Ground  DialogController=POWERSYS.PowerSysDialog  PhysicalDomain=powersysdomain  SubClassName=unknown  LeftPortType=p1  RightPortType=p1  LConnTagsString=a  RConnTagsString=__newr0
  VdcP : PMIOPort  Port=1  Side=Right
  N : PMIOPort  Port=2  Side=Right
  VdcM : PMIOPort  Port=3  Side=Right
  A : PMIOPort  Port=4  Side=Left
  B : PMIOPort  Port=5  Side=Left
  C : PMIOPort  Port=6  Side=Left
  tag scope: Vab_Tr1D=global, Vab_Tr2D=global, Van_Tr1Y=global, Van_Tr2Y=global
  wires:
  Pulses/1 -> Demux/1
  Voltage Measurement/1 -> [Van_Tr1Y]
  Voltage Measurement1/1 -> [Van_Tr2Y]
  Voltage Measurement2/1 -> [Vab_Tr1D]
  Voltage Measurement3/1 -> [Vab_Tr2D]
  Demux/1 -> Three-Level Bridge  1Y/1
  Demux/2 -> Three-Level Bridge  1D/1
  Demux/3 -> Three-Level Bridge  12Y/1
  Demux/4 -> Three-Level Bridge 2D/1
  connections:
  VdcP/RConn1 -- Three-Level Bridge  1Y/RConn1 -- Three-Level Bridge  1D/RConn1 -- Three-Level Bridge  12Y/RConn1 -- Three-Level Bridge 2D/RConn1
  Zigzag transformer Phase-Shifting of +7.5 deg. Tr1Y/RConn2 -- Three-Level Bridge  1Y/LConn2
  Zigzag transformer Phase-Shifting of +7.5 deg. Tr1Y/RConn3 -- Three-Level Bridge  1Y/LConn3
  Zigzag transformer Phase-Shifting of -7.5 deg. Tr2Y/RConn2 -- Three-Level Bridge  12Y/LConn2
  Zigzag transformer Phase-Shifting of -7.5 deg. Tr2Y/RConn3 -- Three-Level Bridge  12Y/LConn3
  Zigzag transformer Phase-Shifting of +7.5 deg. Tr1Y/RConn4 -- Voltage Measurement/LConn2
  Zigzag transformer Phase-Shifting of -7.5 deg. Tr2Y/RConn4 -- Voltage Measurement1/LConn2
  Imes_SH/RConn1 -- Zigzag transformer Phase-Shifting of +7.5 deg. Tr1Y/LConn1
  Imes_SH/RConn2 -- Zigzag transformer Phase-Shifting of +7.5 deg. Tr1Y/LConn2
  Imes_SH/RConn3 -- Zigzag transformer Phase-Shifting of +7.5 deg. Tr1Y/LConn3
  B/RConn1 -- Imes_SH/LConn2
  A/RConn1 -- Imes_SH/LConn1
  C/RConn1 -- Imes_SH/LConn3
  Zigzag transformer Phase-Shifting of +7.5 deg. Tr1Y/LConn4 -- Zigzag transformer Phase-Shifting of +7.5 deg. Tr1Y1/LConn1
  Zigzag transformer Phase-Shifting of +7.5 deg. Tr1Y/LConn5 -- Zigzag transformer Phase-Shifting of +7.5 deg. Tr1Y1/LConn2
  Zigzag transformer Phase-Shifting of +7.5 deg. Tr1Y/LConn6 -- Zigzag transformer Phase-Shifting of +7.5 deg. Tr1Y1/LConn3
  Zigzag transformer Phase-Shifting of +7.5 deg. Tr1Y1/LConn4 -- Zigzag transformer Phase-Shifting of -7.5 deg. Tr2Y/LConn1
  Zigzag transformer Phase-Shifting of +7.5 deg. Tr1Y1/LConn5 -- Zigzag transformer Phase-Shifting of -7.5 deg. Tr2Y/LConn2
  Zigzag transformer Phase-Shifting of +7.5 deg. Tr1Y1/LConn6 -- Zigzag transformer Phase-Shifting of -7.5 deg. Tr2Y/LConn3
  Zigzag transformer Phase-Shifting of -7.5 deg. Tr2Y/LConn4 -- Zigzag transformer Phase-Shifting of -7.5 deg. Tr1Y2/LConn1
  Zigzag transformer Phase-Shifting of -7.5 deg. Tr2Y/LConn5 -- Zigzag transformer Phase-Shifting of -7.5 deg. Tr1Y2/LConn2
  Zigzag transformer Phase-Shifting of -7.5 deg. Tr2Y/LConn6 -- Zigzag transformer Phase-Shifting of -7.5 deg. Tr1Y2/LConn3
  output Ground1/LConn1 -- Zigzag transformer Phase-Shifting of -7.5 deg. Tr1Y2/LConn4 -- Zigzag transformer Phase-Shifting of -7.5 deg. Tr1Y2/LConn5 -- Zigzag transformer Phase-Shifting of -7.5 deg. Tr1Y2/LConn6
  Three-Level Bridge  12Y/RConn3 -- Three-Level Bridge 2D/RConn3 -- VdcM/RConn1 -- Three-Level Bridge  1D/RConn3 -- Three-Level Bridge  1Y/RConn3
  Zigzag transformer Phase-Shifting of +7.5 deg. Tr1Y1/RConn1 -- Three-Level Bridge  1D/LConn1 -- Voltage Measurement2/LConn1
  Zigzag transformer Phase-Shifting of +7.5 deg. Tr1Y1/RConn2 -- Three-Level Bridge  1D/LConn2 -- Voltage Measurement2/LConn2
  Zigzag transformer Phase-Shifting of +7.5 deg. Tr1Y1/RConn3 -- Three-Level Bridge  1D/LConn3
  Three-Level Bridge  12Y/RConn2 -- Three-Level Bridge  1D/RConn2 -- N/RConn1 -- Three-Level Bridge  1Y/RConn2 -- Three-Level Bridge 2D/RConn2
  Zigzag transformer Phase-Shifting of +7.5 deg. Tr1Y/RConn1 -- Three-Level Bridge  1Y/LConn1 -- Voltage Measurement/LConn1
  Zigzag transformer Phase-Shifting of -7.5 deg. Tr2Y/RConn1 -- Three-Level Bridge  12Y/LConn1 -- Voltage Measurement1/LConn1
  Zigzag transformer Phase-Shifting of -7.5 deg. Tr1Y2/RConn1 -- Three-Level Bridge 2D/LConn1 -- Voltage Measurement3/LConn1
  Zigzag transformer Phase-Shifting of -7.5 deg. Tr1Y2/RConn2 -- Three-Level Bridge 2D/LConn2 -- Voltage Measurement3/LConn2
  Zigzag transformer Phase-Shifting of -7.5 deg. Tr1Y2/RConn3 -- Three-Level Bridge 2D/LConn3

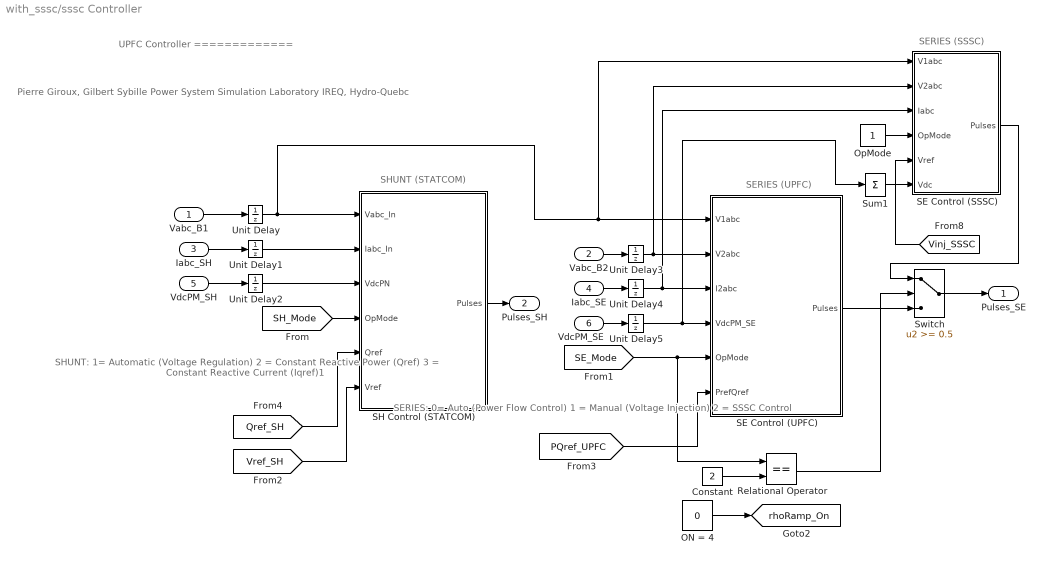
== system with_sssc/sssc Controller ==
  note: Pierre Giroux, Gilbert Sybille
      | Power System Simulation Laboratory
      | IREQ, Hydro-Quebc
  note: SHUNT (STATCOM)
  note: SERIES (UPFC)
  note: UPFC Controller
      | =============
  note: SHUNT:
      | 1= Automatic (Voltage Regulation)
      | 2 = Constant Reactive Power (Qref)
      | 3 = Constant Reactive Current (Iqref)1
  note: SERIES:
      | 0= Auto (Power Flow Control)
      | 1 = Manual (Voltage Injection)
      | 2 = SSSC Control
  note: SERIES (SSSC)
  Vabc_B1 : Inport  PortDimensions=3  OutDataType=sfix(16)  OutScaling=2^0
  Vabc_B2 : Inport  Port=2  PortDimensions=3  OutDataType=sfix(16)  OutScaling=2^0
  "Iabc_SH " : Inport  Port=3  PortDimensions=3  OutDataType=sfix(16)  OutScaling=2^0
  Iabc_SE : Inport  Port=4  PortDimensions=3  OutDataType=sfix(16)  OutScaling=2^0
  "VdcPM_SH " : Inport  Port=5  PortDimensions=2  OutDataType=sfix(16)  OutScaling=2^0
  VdcPM_SE : Inport  Port=6  PortDimensions=2  OutDataType=sfix(16)  OutScaling=2^0
  Constant : Constant  Value=2  OutDataType=sfix(16)  OutScaling=2^0
  ON = 4 : Constant  Value=0  OutDataType=sfix(16)  OutScaling=2^0
  OpMode : Constant  OutDataType=sfix(16)  OutScaling=2^0
  Relational Operator : RelationalOperator  Operator===
  SE Control (SSSC) : Subsystem
  SE Control (UPFC) : Subsystem  mask(Injection Voltage Control){PQref=[8.7 -0.6], Vref_Inj=[0 0], ParK_Vseries=[0.025 1.5*4], Ts=Ts}
      mask prompts: PQref "Reference active and reactive power [ Pref  Qref ] (pu/100MVA):"; Vref_Inj "Manual Voltage Injection: [ Mag(pu)  rho(deg.) ]"; ParK_Vseries "Regulator gain [Kp  Ki ]"; Ts "Sample time:"
      mask init:
      | Kp_Vseries=ParK_Vseries(1);
      | Ki_Vseries=ParK_Vseries(2);
      | Pref=PQref(1);
      | Qref=PQref(2);
      | MagInj=Vref_Inj(1);
      | rhoInj=Vref_Inj(2);
  SH Control (STATCOM) : Subsystem  mask(STATCOM Controller){Vref=1.00, Droop=0.01, Qref1=0, Iqref1=0, ParK_V=[12 3000]*3, ParK_I=[5 40], Ts=Ts}
      mask prompts: Vref "Automatic mode: Voltage setpoint (Vref in pu)"; Droop "Droop (pu/100 MVA):"; Qref1 "Reactive power setpoint (Qref in pu)"; Iqref1 "Reactive Current setpoint (Iqref in pu):"; ParK_V "Voltage regulator gains: [ Kp  Ki ]"; ParK_I "Iq regulator gains: [ Kp  Ki ]"; Ts "Sample time:"
      mask init:
      | Kp_I=ParK_I(1);
      | Ki_I=ParK_I(2);
      | Kp_V=ParK_V(1);
      | Ki_V=ParK_V(2);
  Sum1 : Sum  Inputs=1  OutDataType=sfix(16)  OutScaling=2^0  SaturateOnIntegerOverflow=on  InputSameDT=on  OutDataTypeStr=Inherit: Same as first input
  Switch : Switch  Threshold=0.5  OutDataType=sfix(16)  OutScaling=2^0  SaturateOnIntegerOverflow=on
  Unit Delay{,1..5} (6 alike) : UnitDelay  SampleTime=Ts
  Pulses_SE : Outport  OutDataType=sfix(16)  OutScaling=2^0
  Pulses_SH : Outport  Port=2  OutDataType=sfix(16)  OutScaling=2^0
  tag scope: rhoRamp_On=global
  wires:
  "Iabc_SH "/1 -> Unit Delay1/1
  "VdcPM_SH "/1 -> Unit Delay2/1
  Vabc_B1/1 -> Unit Delay/1
  SH Control (STATCOM)/1(Pulses) -> Pulses_SH/1
  Iabc_SE/1 -> Unit Delay4/1
  Vabc_B2/1 -> Unit Delay3/1
  VdcPM_SE/1 -> Unit Delay5/1
  Unit Delay/1 -> SH Control (STATCOM)/1(Vabc_In), SE Control (UPFC)/1(V1abc), SE Control (SSSC)/1(V1abc)
  Unit Delay1/1 -> SH Control (STATCOM)/2(Iabc_In)
  Unit Delay2/1 -> SH Control (STATCOM)/3(VdcPN)
  Unit Delay3/1 -> SE Control (UPFC)/2(V2abc), SE Control (SSSC)/2(V2abc)
  Unit Delay4/1 -> SE Control (UPFC)/3(I2abc), SE Control (SSSC)/3(Iabc)
  Unit Delay5/1 -> SE Control (UPFC)/4(VdcPM_SE), Sum1/1
  ON = 4/1 -> [rhoRamp_On]
  [SE_Mode] -> SE Control (UPFC)/5(OpMode), Relational Operator/1
  OpMode/1 -> SE Control (SSSC)/4(OpMode)
  [SH_Mode] -> SH Control (STATCOM)/4(OpMode)
  Sum1/1 -> SE Control (SSSC)/6(Vdc)
  Constant/1 -> Relational Operator/2
  [Vref_SH] -> SH Control (STATCOM)/6(Vref)
  [PQref_UPFC] -> SE Control (UPFC)/6(PrefQref)
  [Vinj_SSSC] -> SE Control (SSSC)/5(Vref)
  [Qref_SH] -> SH Control (STATCOM)/5(Qref)
  SE Control (UPFC)/1(Pulses) -> Switch/3
  Switch/1 -> Pulses_SE/1
  SE Control (SSSC)/1(Pulses) -> Switch/1
  Relational Operator/1 -> Switch/2

== system with_sssc/Series Converter/Imes_SE ==
  A->pu : Gain  Gain=500e3*sqrt(3)/100e6/sqrt(2)  ParameterDataType=sfix(16)  ParameterScaling=2^0  OutDataType=sfix(16)  OutScaling=2^0  SaturateOnIntegerOverflow=on  OutDataTypeStr=Inherit: Same as input  ParamDataTypeStr=Inherit: Same as input
  Current Measurement : powerlib/Measurements/Current Measurement  Tag=PoWeRsYsTeMmEaSuReMeNt  DialogController=POWERSYS.PowerSysDialog  SystemSampleTime=-1  PhasorSimulation=off  OutputType=Magnitude  PSBequivalent=0
  Current Measurement1 : powerlib/Measurements/Current Measurement  Tag=PoWeRsYsTeMmEaSuReMeNt  DialogController=POWERSYS.PowerSysDialog  SystemSampleTime=-1  PhasorSimulation=off  OutputType=Magnitude  PSBequivalent=0
  Current Measurement2 : powerlib/Measurements/Current Measurement  Tag=PoWeRsYsTeMmEaSuReMeNt  DialogController=POWERSYS.PowerSysDialog  SystemSampleTime=-1  PhasorSimulation=off  OutputType=Magnitude  PSBequivalent=0
  Mux : Mux  Inputs=3
  "A " : PMIOPort  Port=1  Side=Left
  "B " : PMIOPort  Port=2  Side=Left
  "C " : PMIOPort  Port=3  Side=Left
  " A" : PMIOPort  Port=4  Side=Right
  " B" : PMIOPort  Port=5  Side=Right
  " C" : PMIOPort  Port=6  Side=Right
  tag scope: Iabc_SE=global
  wires:
  Mux/1 -> A->pu/1
  A->pu/1 -> [Iabc_SE]
  Current Measurement/1 -> Mux/1
  Current Measurement2/1 -> Mux/3
  Current Measurement1/1 -> Mux/2
  connections:
  "A "/RConn1 -- Current Measurement/LConn1
  Current Measurement/RConn1 -- " A"/RConn1
  "B "/RConn1 -- Current Measurement1/LConn1
  Current Measurement1/RConn1 -- " B"/RConn1
  "C "/RConn1 -- Current Measurement2/LConn1
  Current Measurement2/RConn1 -- " C"/RConn1

== system with_sssc/Subsystem1/Determine_Qref (STATCOM) ==
  T1 : Inport  OutDataType=sfix(16)  OutScaling=2^0
  T2 : Inport  Port=2  OutDataType=sfix(16)  OutScaling=2^0
  Q1 : Inport  Port=3  OutDataType=sfix(16)  OutScaling=2^0
  Q2 : Inport  Port=4  OutDataType=sfix(16)  OutScaling=2^0
  Constant : Constant  Value=0  OutDataType=sfix(16)  OutScaling=2^0
  Constant1 : Constant  OutDataType=sfix(16)  OutScaling=2^0
  Digital Clock : DigitalClock  SampleTime=Ts
  Multiport Switch : MultiPortSwitch  OutDataType=sfix(16)  OutScaling=2^0  SaturateOnIntegerOverflow=on
  Relational Operator : RelationalOperator  Operator=>
  Relational Operator1 : RelationalOperator  Operator=>
  Sum : Sum  Inputs=+++  OutDataType=sfix(16)  OutScaling=2^0  SaturateOnIntegerOverflow=on
  Qref : Outport  OutDataType=sfix(16)  OutScaling=2^0
  wires:
  Sum/1 -> Multiport Switch/1
  Q2/1 -> Multiport Switch/4
  Q1/1 -> Multiport Switch/3
  Multiport Switch/1 -> Qref/1
  Constant1/1 -> Sum/1
  Relational Operator1/1 -> Sum/3
  Relational Operator/1 -> Sum/2
  Constant/1 -> Multiport Switch/2
  T2/1 -> Relational Operator1/2
  T1/1 -> Relational Operator/2
  Digital Clock/1 -> Relational Operator1/1, Relational Operator/1
